simulink model "TP1_simu_realim_obs"  (R2023b)
settings: Solver=VariableStepAuto  StartTime=0.0  StopTime=10  RelTol=1e-3
values from neighbouring files (symbols this model uses):
  A = Ass    [TP1.m]
  B = Bss    [TP1.m]
  C = Css    [TP1.m]
  D = Dss    [TP1.m]
  Kest = Ka(1:n)    [TP1.m]
  kI = -Ka(end)    [TP1.m]
  Lo = acker(A', C', [-800 -8 -8])'    [TP1.m]
  ue = 4    [TP1.m]
  x1e = 1    [TP1.m]
  x2e = 1    [TP1.m]
  x3e = 0    [TP1.m]
  xeq = [x1e;x2e;x3e]    [TP1.m]
  ye = x2e    (= 1)    [TP1.m]
settings Model: Creator=manuh  LastModifiedBy=ApoloXVIII

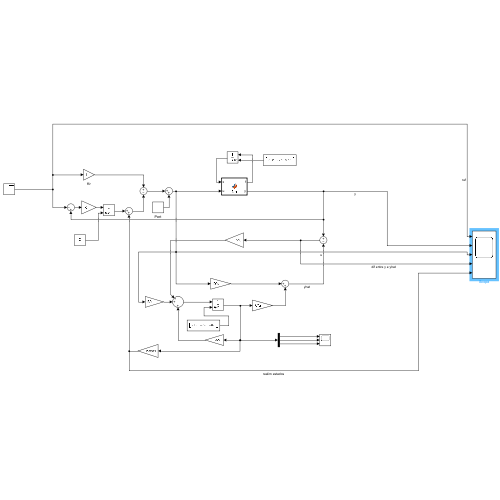
[thumbnail: Simulink's stored preview of the top-level diagram]
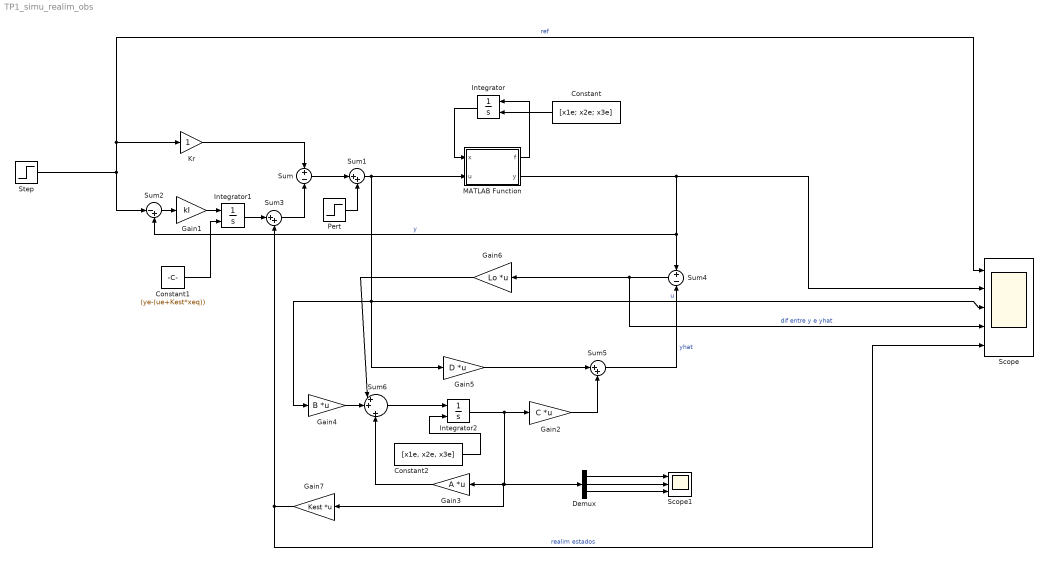
== system TP1_simu_realim_obs ==
  Constant : Constant  Value=[x1e; x2e; x3e]
  Constant1 : Constant  Value=(ye-(ue+Kest*xeq))
  Constant2 : Constant  Value=[x1e, x2e, x3e]
  Demux : Demux  Outputs=3
  Gain1 : Gain  Gain=kI
  Gain2 : Gain  Gain=C  Multiplication=Matrix(K*u)
  Gain3 : Gain  Gain=A  Multiplication=Matrix(K*u)
  Gain4 : Gain  Gain=B  Multiplication=Matrix(K*u)
  Gain5 : Gain  Gain=D  Multiplication=Matrix(K*u)
  Gain6 : Gain  Gain=Lo  Multiplication=Matrix(K*u)
  Gain7 : Gain  Gain=Kest  Multiplication=Matrix(K*u)
  Integrator : Integrator  InitialConditionSource=external
  Integrator1 : Integrator  InitialConditionSource=external
  Integrator2 : Integrator  InitialConditionSource=external
  Kr : Gain
  MATLAB Function : MATLAB Function  TreatAsAtomicUnit=on
  Pert : Step  Time=7  After=0.5  SampleTime=0
  Scope : Scope  NumInputPorts=5
  Scope1 : Scope  NumInputPorts=3
  Step : Step  Time=5  Before=1  After=1.1  SampleTime=0
  Sum : Sum  Inputs=+|-
  Sum1 : Sum  Inputs=|++
  Sum2 : Sum  Inputs=|-+
  Sum3 : Sum  Inputs=|++
  Sum4 : Sum  Inputs=+|-
  Sum5 : Sum  Inputs=|++
  Sum6 : Sum  Inputs=|++|+
  wires:
  Constant/1 -> Integrator/2
  MATLAB Function/1(f) -> Integrator/1
  Integrator/1 -> MATLAB Function/1(x)
  Step/1 -> Scope/1, Kr/1, Sum2/1  "ref"
  Kr/1 -> Sum/1
  Sum2/1 -> Gain1/1
  Gain1/1 -> Integrator1/1
  Integrator1/1 -> Sum3/1
  Sum3/1 -> Sum/2
  Constant1/1 -> Integrator1/2
  Sum1/1 -> Gain4/1, Gain5/1, Scope/3, MATLAB Function/2(u)  "u"
  Pert/1 -> Sum1/2
  Sum4/1 -> Gain6/1, Scope/4  "dif entre y e yhat"
  MATLAB Function/2(y) -> Sum2/2, Sum4/1, Scope/2  "y"
  Gain5/1 -> Sum5/1
  Sum5/1 -> Sum4/2  "yhat"
  Gain2/1 -> Sum5/2
  Integrator2/1 -> Gain7/1, Gain3/1, Demux/1, Gain2/1
  Gain3/1 -> Sum6/3
  Sum6/1 -> Integrator2/1
  Gain4/1 -> Sum6/2
  Gain6/1 -> Sum6/1
  Constant2/1 -> Integrator2/2
  Gain7/1 -> Sum3/2, Scope/5  "realim estados"
  Demux/1 -> Scope1/1
  Demux/2 -> Scope1/2
  Demux/3 -> Scope1/3
  Sum/1 -> Sum1/1

== matlab function TP1_simu_realim_obs/MATLAB Function ==
  data: x input; f output; u input; y output
function [f,y] = fcn(x,u)
%Parámetros del problema
R=4;
L=1e-2;
m=0.1;
g=10;

% Definir funciones de derivadas (f)
f1=u/L-(R/L)*x(1);
f2=x(3);
f3=g-(x(1))/(x(2)*m);

f = [f1; f2; f3];

% Definir la salida y
y=x(2);
